simulink model "obiekt_obserwator_regulatorStanObserwowany"  (R2024b)
settings: Solver=ode23s  StartTime=0.0  StopTime=3  RelTol=1e-3
values from neighbouring files (symbols this model uses):
  K = acker(A, B, [s_b s_b s_b s_b])    [parametry_obserwator_regulator.m]    (also in parametry_regulator_calkowy.m = KK_e(1, 1:n))
  obs1 = -10    [wykresy_obserwator_stan_obserwowany.m]
  obs2 = 10    [wykresy_obserwator_stan_obserwowany.m]
  obs3 = -20    [wykresy_obserwator_stan_obserwowany.m]
  obs4 = 20    [wykresy_obserwator_stan_obserwowany.m]
undefined symbols (not defined in the file or in its folder): L1, L2, L3, L4
settings Model: Creator=mparadow  LastModifiedBy=mparadow

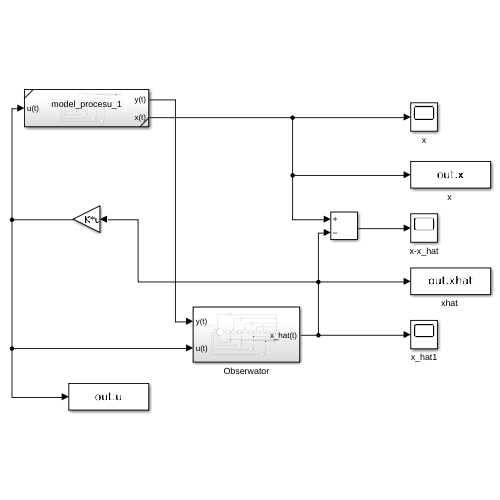
[thumbnail: Simulink's stored preview of the top-level diagram]
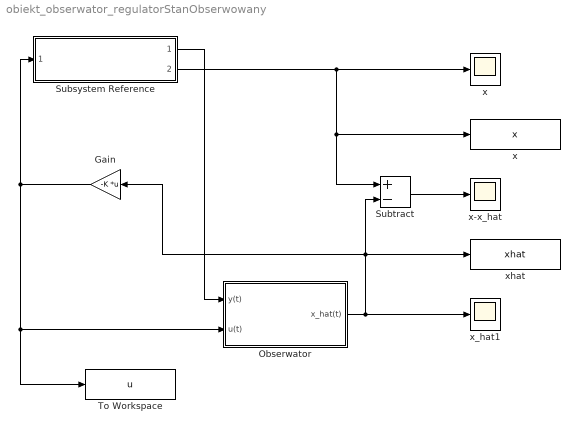
== system obiekt_obserwator_regulatorStanObserwowany ==
  Gain : Gain  Gain=-K  Multiplication=Matrix(K*u)
  Obserwator : Subsystem
  Subsystem Reference : Subsystem  ReferencedSubsystem=model_procesu_1
  Subtract : Sum  Inputs=+-
  To Workspace : ToWorkspace  VariableName=u  SaveFormat=Structure With Time  SampleTime=-1
  x : Scope
  "x " : ToWorkspace  VariableName=x  SaveFormat=Structure With Time  SampleTime=-1
  x-x_hat : Scope
  x_hat1 : Scope
  "xhat " : ToWorkspace  VariableName=xhat  SaveFormat=Structure With Time  SampleTime=-1
  wires:
  Gain/1 -> To Workspace/1, Obserwator/2(u(t)), Subsystem Reference/1
  Subsystem Reference/1 -> Obserwator/1(y(t))
  Obserwator/1(x_hat(t)) -> "xhat "/1, Subtract/2, Gain/1, x_hat1/1
  Subtract/1 -> x-x_hat/1
  Subsystem Reference/2 -> "x "/1, Subtract/1, x/1

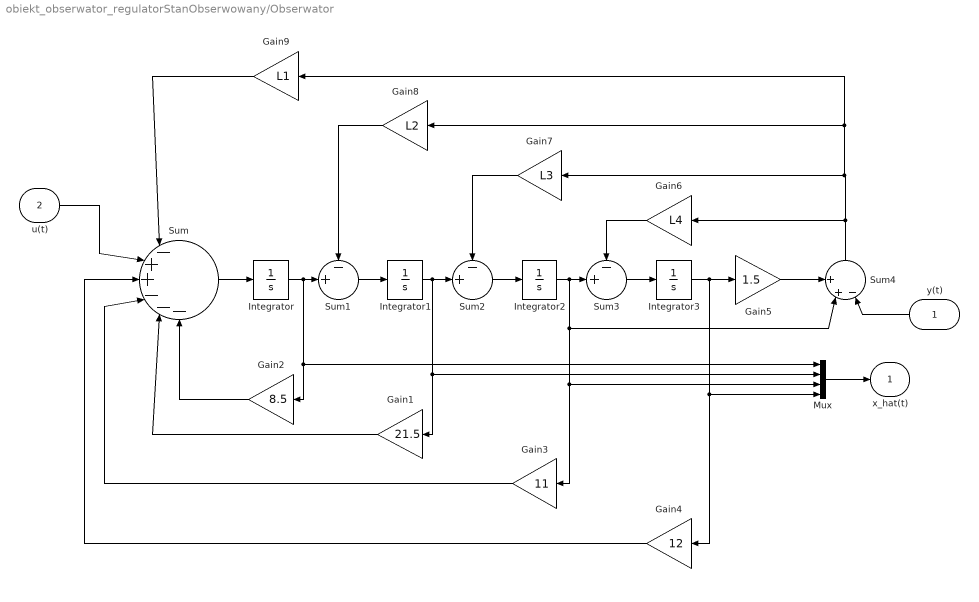
== system obiekt_obserwator_regulatorStanObserwowany/Obserwator ==
  y(t) : Inport
  u(t) : Inport  Port=2
  Gain1 : Gain  Gain=21.5
  Gain2 : Gain  Gain=8.5
  Gain3 : Gain  Gain=11
  Gain4 : Gain  Gain=12
  Gain5 : Gain  Gain=1.5
  Gain6 : Gain  Gain=L4
  Gain7 : Gain  Gain=L3
  Gain8 : Gain  Gain=L2
  Gain9 : Gain  Gain=L1
  Integrator : Integrator  InitialCondition=obs1
  Integrator1 : Integrator  InitialCondition=obs2
  Integrator2 : Integrator  InitialCondition=obs3
  Integrator3 : Integrator  InitialCondition=obs4
  Mux : Mux
  Sum : Sum  Inputs=|-++---
  Sum1 : Sum  Inputs=-+|
  Sum2 : Sum  Inputs=-+|
  Sum3 : Sum  Inputs=-+|
  Sum4 : Sum  Inputs=++-|
  x_hat(t) : Outport
  wires:
  Integrator/1 -> Sum1/2, Mux/1, Gain2/1
  Integrator2/1 -> Sum3/2, Sum4/2, Mux/3, Gain3/1
  Sum/1 -> Integrator/1
  Gain2/1 -> Sum/6
  Integrator1/1 -> Sum2/2, Mux/2, Gain1/1
  Sum1/1 -> Integrator1/1
  Gain1/1 -> Sum/5
  Gain3/1 -> Sum/4
  Sum3/1 -> Integrator3/1
  Integrator3/1 -> Gain5/1, Mux/4, Gain4/1
  Gain4/1 -> Sum/3
  u(t)/1 -> Sum/2
  Sum2/1 -> Integrator2/1
  Mux/1 -> x_hat(t)/1
  Gain5/1 -> Sum4/1
  y(t)/1 -> Sum4/3
  Sum4/1 -> Gain9/1, Gain8/1, Gain7/1, Gain6/1
  Gain6/1 -> Sum3/1
  Gain7/1 -> Sum2/1
  Gain8/1 -> Sum1/1
  Gain9/1 -> Sum/1
